simulink library "scp"  (R2021b)
settings: Solver=VariableStepAuto  StartTime=0.0  StopTime=10.0  RelTol=1e-3
undefined symbols (not defined in the file or in its folder): ENUM_ABSACTIVE_ACTIVE, ENUM_ABSACTIVE_INACTIVE, ENUM_ABSFAILED_FAILED, ENUM_ABSFAILED_NORMAL, ENUM_ABSFULLYOPER_FULLYOPER, ENUM_ABSFULLYOPER_INVALID, ENUM_ABSFULLYOPER_NOTFULLYOPER, ENUM_ABSFULLYOPER_RESERVED, ENUM_ABSWNLMPSTA_CONSTANT, ENUM_ABSWNLMPSTA_OFF, ENUM_AMBERWNLMPSTA_CONSTANT, ENUM_AMBERWNLMPSTA_OFF, ENUM_ANTILBRAKABSACT_ACTIVE, ENUM_ANTILBRAKABSACT_INVALID, ENUM_ANTILBRAKABSACT_PASSIVE, ENUM_ANTILBRAKABSACT_RESERVED, ENUM_BRKSWSTA_ACTIVE, ENUM_BRKSWSTA_INACTIVE, ENUM_EBSAMWARNLAMPSTA_NOACTION, ENUM_EBSAMWARNLAMPSTA_OFF, ENUM_EBSAMWARNLAMPSTA_ON, ENUM_EBSAMWARNLAMPSTA_RESERVED, ENUM_EBSBRAKESW_ERROR, ENUM_EBSBRAKESW_INVALID, ENUM_EBSBRAKESW_PRESSED, ENUM_EBSBRAKESW_UNPRESSED, ENUM_EBSREDWARNLAMPSTA_NOACTION, ENUM_EBSREDWARNLAMPSTA_OFF, ENUM_EBSREDWARNLAMPSTA_ON, ENUM_EBSREDWARNLAMPSTA_RESERVED, ENUM_FRDOORPOSISTA_CLOSED, ENUM_FRDOORPOSISTA_NODEFINE, ENUM_FRDOORPOSISTA_OPEN, ENUM_FRDOORPOSISTA_PARTIALOPEN, ENUM_HILLHOLDERMODE_ACTIVE, ENUM_HILLHOLDERMODE_ACTIVE2INACTIVE, ENUM_HILLHOLDERMODE_ACTIVEMAYPARK, ENUM_HILLHOLDERMODE_INACTIVE, ENUM_HILLHOLDERMODE_INVALID, ENUM_HILLHOLDERMODE_NOFUNC, ENUM_HILLHOLDERMODE_RESERVED4, ENUM_HILLHOLDERMODE_RESERVED5, ENUM_HSAACTIVE_ACTIVE, ENUM_HSAACTIVE_INACTIVE, ENUM_HSAFAILED_FAILED, ENUM_HSAFAILED_NORMAL, ENUM_OPENSTATUSOFDOOR1_CLOSED, ENUM_OPENSTATUSOFDOOR1_OPENED, ENUM_REDWNLMPSTA_CONSTANT, ENUM_REDWNLMPSTA_OFF, FALSE, KSCP_DelayECBAMandECDT_s, KSCP_DelayECDTandECDT_s, KSCP_DelayECDTandRCBAM_s, KSCP_DelayRCBAMandRCDT_s, KSCP_DelayRCDTandECBAM_s, KSCP_DelayRCDTandRCDT_s, KTQD_MCUMaxRefTq_Nm, TRUE
libraries: FVT_lib x14, hcu_lib x10, simulink x2
settings Model: Creator=FVT23118  LastModifiedBy=FVT22063

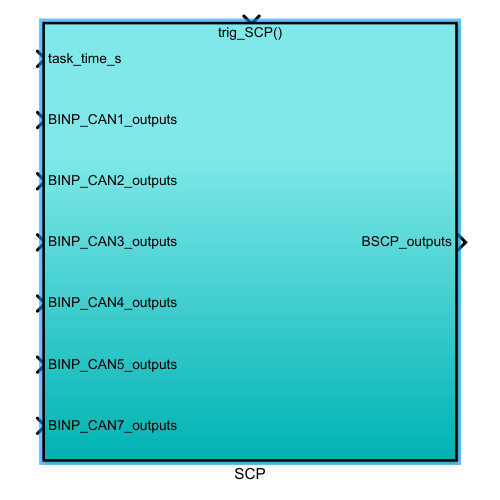
[thumbnail: Simulink's stored preview of the top-level diagram]
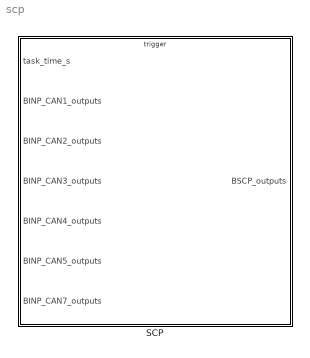
== system scp ==
  SCP : Subsystem
      settings: RTWSystemCode=Nonreusable function  RTWFcnNameOpts=Use subsystem name  RTWFileNameOpts=Use subsystem name

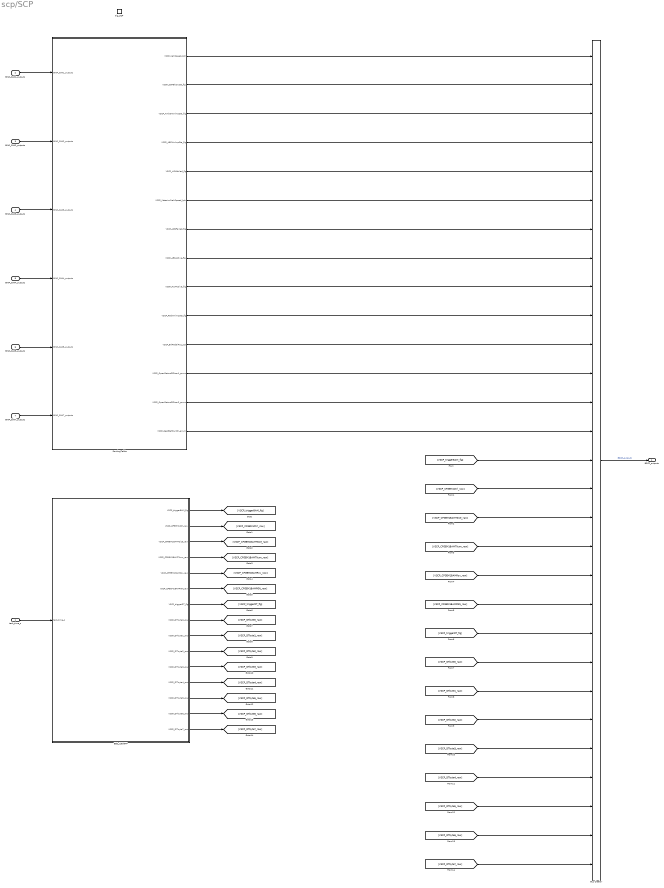
== system scp/SCP ==
  task_time_s : Inport
  BINP_CAN1_outputs : Inport  Port=2  OutDataTypeStr=Bus: BINP_CAN1_outputs
  BINP_CAN2_outputs : Inport  Port=3  OutDataTypeStr=Bus: BINP_CAN2_outputs
  BINP_CAN3_outputs : Inport  Port=4  OutDataTypeStr=Bus: BINP_CAN3_outputs
  BINP_CAN4_outputs : Inport  Port=5  OutDataTypeStr=Bus: BINP_CAN4_outputs
  BINP_CAN5_outputs : Inport  Port=6  OutDataTypeStr=Bus: BINP_CAN5_outputs
  BINP_CAN7_outputs : Inport  Port=7  OutDataTypeStr=Bus: BINP_CAN7_outputs
  trig_SCP : TriggerPort  TriggerType=function-call  VariantControl=(inherit)  PortDimensions=1
  Bus Creator : BusCreator  Inputs=29  OutDataTypeStr=Bus: BSCP_outputs  NonVirtualBus=on
  EBS_J1939TP : Subsystem
  RoutingTable : Subsystem
  BSCP_outputs : Outport  OutDataTypeStr=Bus: BSCP_outputs
  wires:
  BINP_CAN1_outputs/1 -> RoutingTable/1(BINP_CAN1_outputs)
  BINP_CAN4_outputs/1 -> RoutingTable/4(BINP_CAN4_outputs)
  BINP_CAN3_outputs/1 -> RoutingTable/3(BINP_CAN3_outputs)
  BINP_CAN2_outputs/1 -> RoutingTable/2(BINP_CAN2_outputs)
  BINP_CAN5_outputs/1 -> RoutingTable/5(BINP_CAN5_outputs)
  BINP_CAN7_outputs/1 -> RoutingTable/6(BINP_CAN7_outputs)
  RoutingTable/5(VSCP_HSAFailed_flg) -> Bus Creator/5
  RoutingTable/6(VSCP_MeterIndVehSpeed_kph) -> Bus Creator/6
  RoutingTable/4(VSCP_ABSWnlmpSta_flg) -> Bus Creator/4
  RoutingTable/7(VSCP_ABSFailed_flg) -> Bus Creator/7
  RoutingTable/3(VSCP_AmberWnlmpSta_flg) -> Bus Creator/3
  RoutingTable/8(VSCP_ABSActive_flg) -> Bus Creator/8
  RoutingTable/2(VSCP_SCPBrkSwSta_flg) -> Bus Creator/2
  RoutingTable/9(VSCP_HSAActive_flg) -> Bus Creator/9
  RoutingTable/1(VSCP_VehSpeed_kph) -> Bus Creator/1
  RoutingTable/10(VSCP_RedWnlmpSta_flg) -> Bus Creator/10
  RoutingTable/11(VSCP_BrkPedalPos_pct) -> Bus Creator/11
  RoutingTable/12(VSCP_OpenStatusOfDoor1_enum) -> Bus Creator/12
  RoutingTable/13(VSCP_OpenStatusOfDoor2_enum) -> Bus Creator/13
  RoutingTable/14(VSCP_SeatBeltSwitch_enum) -> Bus Creator/14
  Bus Creator/1 -> BSCP_outputs/1  "BSCP_outputs"
  EBS_J1939TP/1(VSCP_triggerBAM_flg) -> [VSCP_triggerBAM_flg]
  EBS_J1939TP/2(VSCP_CFGEM1Ctrl_raw) -> [VSCP_CFGEM1Ctrl_raw]
  EBS_J1939TP/3(VSCP_CFGEM1BAMTSize_raw) -> [VSCP_CFGEM1BAMTSize_raw]
  EBS_J1939TP/4(VSCP_CFGEM1BAMTNum_raw) -> [VSCP_CFGEM1BAMTNum_raw]
  EBS_J1939TP/5(VSCP_CFGEM1BAMRsv_raw) -> [VSCP_CFGEM1BAMRsv_raw]
  EBS_J1939TP/6(VSCP_CFGEM1BAMPGN_raw) -> [VSCP_CFGEM1BAMPGN_raw]
  EBS_J1939TP/7(VSCP_triggerDT_flg) -> [VSCP_triggerDT_flg]
  EBS_J1939TP/8(VSCP_DTbyte0_raw) -> [VSCP_DTbyte0_raw]
  EBS_J1939TP/9(VSCP_DTbyte1_raw) -> [VSCP_DTbyte1_raw]
  EBS_J1939TP/10(VSCP_DTbyte2_raw) -> [VSCP_DTbyte2_raw]
  EBS_J1939TP/11(VSCP_DTbyte3_raw) -> [VSCP_DTbyte3_raw]
  EBS_J1939TP/12(VSCP_DTbyte4_raw) -> [VSCP_DTbyte4_raw]
  EBS_J1939TP/13(VSCP_DTbyte5_raw) -> [VSCP_DTbyte5_raw]
  EBS_J1939TP/14(VSCP_DTbyte6_raw) -> [VSCP_DTbyte6_raw]
  EBS_J1939TP/15(VSCP_DTbyte7_raw) -> [VSCP_DTbyte7_raw]
  [VSCP_DTbyte7_raw] -> Bus Creator/29
  [VSCP_DTbyte6_raw] -> Bus Creator/28
  [VSCP_DTbyte5_raw] -> Bus Creator/27
  [VSCP_DTbyte4_raw] -> Bus Creator/26
  [VSCP_DTbyte3_raw] -> Bus Creator/25
  [VSCP_DTbyte2_raw] -> Bus Creator/24
  [VSCP_DTbyte1_raw] -> Bus Creator/23
  [VSCP_DTbyte0_raw] -> Bus Creator/22
  [VSCP_triggerDT_flg] -> Bus Creator/21
  [VSCP_CFGEM1BAMPGN_raw] -> Bus Creator/20
  [VSCP_CFGEM1BAMRsv_raw] -> Bus Creator/19
  [VSCP_CFGEM1BAMTNum_raw] -> Bus Creator/18
  [VSCP_CFGEM1BAMTSize_raw] -> Bus Creator/17
  [VSCP_CFGEM1Ctrl_raw] -> Bus Creator/16
  [VSCP_triggerBAM_flg] -> Bus Creator/15
  task_time_s/1 -> EBS_J1939TP/1(task_time_s)

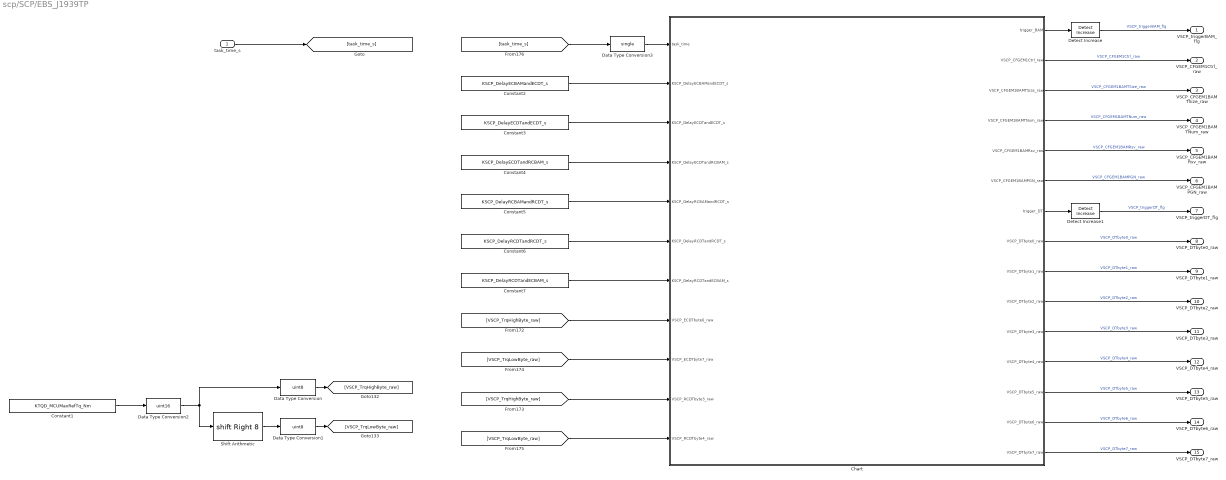
== system scp/SCP/EBS_J1939TP ==
  task_time_s : Inport
  Chart : Stateflow chart  TreatAsAtomicUnit=on
  Constant1 : Constant  Value=KTQD_MCUMaxRefTq_Nm
  Constant2 : Constant  Value=KSCP_DelayECBAMandECDT_s
  Constant3 : Constant  Value=KSCP_DelayECDTandECDT_s
  Constant4 : Constant  Value=KSCP_DelayECDTandRCBAM_s
  Constant5 : Constant  Value=KSCP_DelayRCBAMandRCDT_s
  Constant6 : Constant  Value=KSCP_DelayRCDTandRCDT_s
  Constant7 : Constant  Value=KSCP_DelayRCDTandECBAM_s
  Data Type Conversion : DataTypeConversion  OutDataTypeStr=uint8
  Data Type Conversion1 : DataTypeConversion  OutDataTypeStr=uint8
  Data Type Conversion2 : DataTypeConversion  OutDataTypeStr=uint16
  Data Type Conversion3 : DataTypeConversion  OutDataTypeStr=single
  Detect Increase : simulink/Logic and Bit Operations/Detect Increase  vinit=0.0  OutDataTypeStr=boolean
  Detect Increase1 : simulink/Logic and Bit Operations/Detect Increase  vinit=0.0  OutDataTypeStr=boolean
  Shift Arithmetic : ArithShift  BitShiftNumber=8  BitShiftDirection=Right
  VSCP_triggerBAM_flg : Outport
  VSCP_CFGEM1Ctrl_raw : Outport  Port=2
  VSCP_CFGEM1BAMTSize_raw : Outport  Port=3
  VSCP_CFGEM1BAMTNum_raw : Outport  Port=4
  VSCP_CFGEM1BAMRsv_raw : Outport  Port=5
  VSCP_CFGEM1BAMPGN_raw : Outport  Port=6
  VSCP_triggerDT_flg : Outport  Port=7
  VSCP_DTbyte0_raw : Outport  Port=8
  VSCP_DTbyte1_raw : Outport  Port=9
  VSCP_DTbyte2_raw : Outport  Port=10
  VSCP_DTbyte3_raw : Outport  Port=11
  VSCP_DTbyte4_raw : Outport  Port=12
  VSCP_DTbyte5_raw : Outport  Port=13
  VSCP_DTbyte6_raw : Outport  Port=14
  VSCP_DTbyte7_raw : Outport  Port=15
  wires:
  Constant2/1 -> Chart/2(KSCP_DelayECBAMandECDT_s)
  [task_time_s] -> Data Type Conversion3/1
  Data Type Conversion1/1 -> [VSCP_TrqLowByte_raw]
  [VSCP_TrqHighByte_raw] -> Chart/10(VSCP_RCDTbyte3_raw)
  [VSCP_TrqHighByte_raw] -> Chart/8(VSCP_ECDTbyte6_raw)
  Constant4/1 -> Chart/4(KSCP_DelayECDTandRCBAM_s)
  [VSCP_TrqLowByte_raw] -> Chart/11(VSCP_RCDTbyte4_raw)
  Constant1/1 -> Data Type Conversion2/1
  Constant5/1 -> Chart/5(KSCP_DelayRCBAMandRCDT_s)
  Data Type Conversion2/1 -> Data Type Conversion/1, Shift Arithmetic/1
  Shift Arithmetic/1 -> Data Type Conversion1/1
  Constant3/1 -> Chart/3(KSCP_DelayECDTandECDT_s)
  Constant6/1 -> Chart/6(KSCP_DelayRCDTandRCDT_s)
  Data Type Conversion/1 -> [VSCP_TrqHighByte_raw]
  [VSCP_TrqLowByte_raw] -> Chart/9(VSCP_ECDTbyte7_raw)
  Constant7/1 -> Chart/7(KSCP_DelayRCDTandECBAM_s)
  Chart/1(trigger_BAM) -> Detect Increase/1
  Chart/7(trigger_DT) -> Detect Increase1/1
  Detect Increase/1 -> VSCP_triggerBAM_flg/1  "VSCP_triggerBAM_flg"
  Chart/2(VSCP_CFGEM1Ctrl_raw) -> VSCP_CFGEM1Ctrl_raw/1  "VSCP_CFGEM1Ctrl_raw"
  Chart/3(VSCP_CFGEM1BAMTSize_raw) -> VSCP_CFGEM1BAMTSize_raw/1  "VSCP_CFGEM1BAMTSize_raw"
  Chart/4(VSCP_CFGEM1BAMTNum_raw) -> VSCP_CFGEM1BAMTNum_raw/1  "VSCP_CFGEM1BAMTNum_raw"
  Chart/5(VSCP_CFGEM1BAMRsv_raw) -> VSCP_CFGEM1BAMRsv_raw/1  "VSCP_CFGEM1BAMRsv_raw"
  Chart/6(VSCP_CFGEM1BAMPGN_raw) -> VSCP_CFGEM1BAMPGN_raw/1  "VSCP_CFGEM1BAMPGN_raw"
  Detect Increase1/1 -> VSCP_triggerDT_flg/1  "VSCP_triggerDT_flg"
  Chart/8(VSCP_DTbyte0_raw) -> VSCP_DTbyte0_raw/1  "VSCP_DTbyte0_raw"
  Chart/9(VSCP_DTbyte1_raw) -> VSCP_DTbyte1_raw/1  "VSCP_DTbyte1_raw"
  Chart/10(VSCP_DTbyte2_raw) -> VSCP_DTbyte2_raw/1  "VSCP_DTbyte2_raw"
  Chart/11(VSCP_DTbyte3_raw) -> VSCP_DTbyte3_raw/1  "VSCP_DTbyte3_raw"
  Chart/12(VSCP_DTbyte4_raw) -> VSCP_DTbyte4_raw/1  "VSCP_DTbyte4_raw"
  Chart/13(VSCP_DTbyte5_raw) -> VSCP_DTbyte5_raw/1  "VSCP_DTbyte5_raw"
  Chart/14(VSCP_DTbyte6_raw) -> VSCP_DTbyte6_raw/1  "VSCP_DTbyte6_raw"
  Chart/15(VSCP_DTbyte7_raw) -> VSCP_DTbyte7_raw/1  "VSCP_DTbyte7_raw"
  task_time_s/1 -> [task_time_s]
  Data Type Conversion3/1 -> Chart/1(task_time)

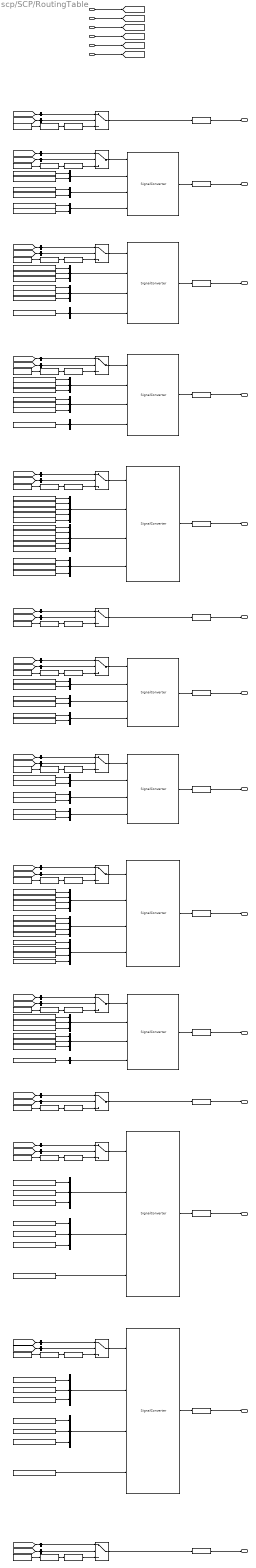
== system scp/SCP/RoutingTable ==
  BINP_CAN1_outputs : Inport
  BINP_CAN2_outputs : Inport  Port=2
  BINP_CAN3_outputs : Inport  Port=3
  BINP_CAN4_outputs : Inport  Port=4
  BINP_CAN5_outputs : Inport  Port=5
  BINP_CAN7_outputs : Inport  Port=6
  Constant : Constant  Value=ENUM_EBSBRAKESW_UNPRESSED
  Constant1 : Constant  Value=ENUM_EBSBRAKESW_PRESSED
  Constant10 : Constant  Value=ENUM_ABSFULLYOPER_RESERVED
  Constant11 : Constant  Value=ENUM_ABSWNLMPSTA_OFF
  Constant12 : Constant  Value=ENUM_ABSFULLYOPER_INVALID
  Constant13 : Constant  Value=ENUM_ABSWNLMPSTA_OFF
  Constant14 : Constant  Value=ENUM_AMBERWNLMPSTA_OFF
  Constant15 : Constant  Value=ENUM_EBSAMWARNLAMPSTA_NOACTION
  Constant16 : Constant  Value=ENUM_AMBERWNLMPSTA_CONSTANT
  Constant17 : Constant  Value=ENUM_EBSAMWARNLAMPSTA_OFF
  Constant18 : Constant  Value=ENUM_EBSAMWARNLAMPSTA_ON
  Constant19 : Constant  Value=ENUM_AMBERWNLMPSTA_OFF
  Constant2 : Constant  Value=ENUM_BRKSWSTA_INACTIVE
  Constant20 : Constant  Value=ENUM_HILLHOLDERMODE_RESERVED4
  Constant{21,23,26,29} (4 alike) : Constant  Value=ENUM_HSAFAILED_NORMAL
  Constant22 : Constant  Value=ENUM_HILLHOLDERMODE_ACTIVE2INACTIVE
  Constant24 : Constant  Value=ENUM_HILLHOLDERMODE_INACTIVE
  Constant25 : Constant  Value=ENUM_HILLHOLDERMODE_ACTIVE
  Constant27 : Constant  Value=ENUM_HILLHOLDERMODE_NOFUNC
  Constant28 : Constant  Value=ENUM_HILLHOLDERMODE_ACTIVEMAYPARK
  Constant3 : Constant  Value=ENUM_BRKSWSTA_ACTIVE
  Constant30 : Constant  Value=ENUM_HSAFAILED_FAILED
  Constant31 : Constant  Value=ENUM_HILLHOLDERMODE_RESERVED5
  Constant32 : Constant  Value=ENUM_HILLHOLDERMODE_INVALID
  Constant33 : Constant  Value=ENUM_ABSFULLYOPER_RESERVED
  Constant34 : Constant  Value=ENUM_ABSFULLYOPER_INVALID
  Constant35 : Constant  Value=ENUM_ANTILBRAKABSACT_RESERVED
  Constant36 : Constant  Value=ENUM_ABSFAILED_NORMAL
  Constant37 : Constant  Value=ENUM_ABSFULLYOPER_NOTFULLYOPER
  Constant38 : Constant  Value=ENUM_ABSFULLYOPER_FULLYOPER
  Constant39 : Constant  Value=ENUM_ABSFAILED_FAILED
  Constant4 : Constant  Value=ENUM_EBSBRAKESW_ERROR
  Constant40 : Constant  Value=ENUM_ANTILBRAKABSACT_INVALID
  Constant41 : Constant  Value=ENUM_ABSACTIVE_ACTIVE
  Constant42 : Constant  Value=ENUM_ANTILBRAKABSACT_PASSIVE
  Constant43 : Constant  Value=ENUM_ANTILBRAKABSACT_ACTIVE
  Constant44 : Constant  Value=ENUM_ABSACTIVE_INACTIVE
  Constant45 : Constant  Value=ENUM_HILLHOLDERMODE_RESERVED4
  Constant46 : Constant  Value=ENUM_HSAACTIVE_INACTIVE
  Constant47 : Constant  Value=ENUM_HILLHOLDERMODE_ACTIVE2INACTIVE
  Constant48 : Constant  Value=ENUM_HSAACTIVE_ACTIVE
  Constant49 : Constant  Value=ENUM_HILLHOLDERMODE_INACTIVE
  Constant5 : Constant  Value=ENUM_EBSBRAKESW_INVALID
  Constant50 : Constant  Value=ENUM_HILLHOLDERMODE_ACTIVE
  Constant51 : Constant  Value=ENUM_HSAACTIVE_ACTIVE
  Constant52 : Constant  Value=ENUM_HILLHOLDERMODE_NOFUNC
  Constant53 : Constant  Value=ENUM_HILLHOLDERMODE_ACTIVEMAYPARK
  Constant54 : Constant  Value=ENUM_HSAACTIVE_ACTIVE
  Constant55 : Constant  Value=ENUM_EBSREDWARNLAMPSTA_RESERVED
  Constant56 : Constant  Value=ENUM_HILLHOLDERMODE_RESERVED5
  Constant57 : Constant  Value=ENUM_HILLHOLDERMODE_INVALID
  Constant58 : Constant  Value=ENUM_EBSREDWARNLAMPSTA_NOACTION
  Constant59 : Constant  Value=ENUM_REDWNLMPSTA_CONSTANT
  Constant6 : Constant  Value=ENUM_ABSFULLYOPER_NOTFULLYOPER
  Constant60 : Constant  Value=ENUM_EBSREDWARNLAMPSTA_OFF
  Constant61 : Constant  Value=ENUM_EBSREDWARNLAMPSTA_ON
  Constant62 : Constant  Value=ENUM_REDWNLMPSTA_OFF
  Constant63 : Constant  Value=ENUM_REDWNLMPSTA_OFF
  Constant64 : Constant  Value=ENUM_FRDOORPOSISTA_NODEFINE
  Constant65 : Constant  Value=ENUM_OPENSTATUSOFDOOR1_CLOSED
  Constant66 : Constant  Value=ENUM_FRDOORPOSISTA_PARTIALOPEN
  Constant{67,70,74,77} (4 alike) : Constant  Value=ENUM_OPENSTATUSOFDOOR1_OPENED
  Constant68 : Constant  Value=ENUM_FRDOORPOSISTA_CLOSED
  Constant69 : Constant  Value=ENUM_FRDOORPOSISTA_OPEN
  Constant7 : Constant  Value=ENUM_ABSFULLYOPER_FULLYOPER
  Constant71 : Constant  Value=ENUM_FRDOORPOSISTA_NODEFINE
  Constant72 : Constant  Value=ENUM_OPENSTATUSOFDOOR1_CLOSED
  Constant73 : Constant  Value=ENUM_FRDOORPOSISTA_PARTIALOPEN
  Constant75 : Constant  Value=ENUM_FRDOORPOSISTA_CLOSED
  Constant76 : Constant  Value=ENUM_FRDOORPOSISTA_OPEN
  Constant8 : Constant  Value=ENUM_EBSAMWARNLAMPSTA_RESERVED
  Constant9 : Constant  Value=ENUM_ABSWNLMPSTA_CONSTANT
  Mux{,1..2,12..17} (9 alike) : Mux  Inputs=2
  Mux10 : Mux  Inputs=5
  Mux{3..4,6..7,11,21,23..27} (11 alike) : Mux  Inputs=3
  Mux18 : Mux
  Mux19 : Mux
  Mux20 : Mux
  Mux22 : Mux  Inputs=1
  Mux5 : Mux  Inputs=1
  Mux8 : Mux  Inputs=1
  Mux9 : Mux  Inputs=5
  SignalConverter{1..3,5..6,8} (6 alike) : hcu_lib/Basic_Blocks/SignalConverter  SourceSignalInitialValue=0  SourceSignalUpperLimit=3  SourceSignalLowerLimit=0  ConvertedSignalInitialValue=0
  SignalConverter10 : hcu_lib/Basic_Blocks/SignalConverter  SourceSignalInitialValue=0  SourceSignalUpperLimit=15  SourceSignalLowerLimit=0  ConvertedSignalInitialValue=0
  SignalConverter4 : hcu_lib/Basic_Blocks/SignalConverter  SourceSignalInitialValue=0  SourceSignalUpperLimit=7  SourceSignalLowerLimit=0  ConvertedSignalInitialValue=0
  SignalConverter7 : hcu_lib/Basic_Blocks/SignalConverter  SourceSignalInitialValue=0  SourceSignalUpperLimit=7  SourceSignalLowerLimit=0  ConvertedSignalInitialValue=0
  SignalConverter9 : hcu_lib/Basic_Blocks/SignalConverter  SourceSignalInitialValue=0  SourceSignalUpperLimit=15  SourceSignalLowerLimit=0  ConvertedSignalInitialValue=0
  convert{1,4,11..12,21..22} (6 alike) : DataTypeConversion  OutDataTypeStr=single
  convert{3,6,8,10,14,16..17,20,27} (9 alike) : DataTypeConversion  OutDataTypeStr=boolean
  convert{2,5,7,9,13,15,18..19,23..26,28} (13 alike) : DataTypeConversion  OutDataTypeStr=uint8
  convert_in : FVT_lib/hal/convert_in  gain=0.00390625  offset=0
  convert_in{1..4,6..9,11..13} (11 alike) : FVT_lib/hal/convert_in  gain=1  offset=0
  convert_in10 : FVT_lib/hal/convert_in  gain=0.4  offset=0
  convert_in5 : FVT_lib/hal/convert_in  gain=0.00390625  offset=0
  cst_1 : Constant  Value=0xFB00
  cst_{2..5,7..11,14} (10 alike) : Constant  Value=0x0
  cst_12 : Constant  Value=0x3
  cst_13 : Constant  Value=0x3
  cst_6 : Constant  Value=0xFB00
  slr2_1 : BusSelector  OutputSignals=VINP_CANMsgValidEBC2_flg
  slr2_{2..4,7..8,10..11} (7 alike) : BusSelector  OutputSignals=VINP_CANMsgValidEBC1_flg
  slr2_12 : BusSelector  OutputSignals=VINP_CANMsgValidDoorFr1_flg
  slr2_13 : BusSelector  OutputSignals=VINP_CANMsgValidDoorFr1_flg
  slr2_14 : BusSelector  OutputSignals=VINP_CANMsgValidZ24CE1000_flg
  slr2_5 : BusSelector  OutputSignals=VINP_CANMsgValidEBC5_flg
  slr2_6 : BusSelector  OutputSignals=VINP_CANMsgValidEBC2_flg
  slr2_9 : BusSelector  OutputSignals=VINP_CANMsgValidEBC5_flg
  slr_1 : BusSelector  OutputSignals=VINP_FASpeed_kph
  slr_10 : BusSelector  OutputSignals=VINP_EBSRedWarnLampSta_enum
  slr_11 : BusSelector  OutputSignals=VINP_BrakePedalPos_pct
  slr_12 : BusSelector  OutputSignals=VINP_DoorFrDoorpositionsta_enum
  slr_13 : BusSelector  OutputSignals=VINP_DoorFrDoorpositionsta_enum
  slr_14 : BusSelector  OutputSignals=VINP_Z24BCMSeatBeltSWSta_flg
  slr_2 : BusSelector  OutputSignals=VINP_EBSBrakeSw_enum
  slr_3 : BusSelector  OutputSignals=VINP_EBSAmWarnLampSta_enum
  slr_4 : BusSelector  OutputSignals=VINP_ABSFullyOper_enum
  slr_5 : BusSelector  OutputSignals=VINP_HillHolderMode_enum
  slr_6 : BusSelector  OutputSignals=VINP_FASpeed_kph
  slr_7 : BusSelector  OutputSignals=VINP_ABSFullyOper_enum
  slr_8 : BusSelector  OutputSignals=VINP_AntiLBrakABSAct_enum
  slr_9 : BusSelector  OutputSignals=VINP_HillHolderMode_enum
  sw_{1..14} (14 alike) : Switch  Criteria=u2 > Threshold
  VSCP_VehSpeed_kph : Outport
  VSCP_SCPBrkSwSta_flg : Outport  Port=2
  VSCP_AmberWnlmpSta_flg : Outport  Port=3
  VSCP_ABSWnlmpSta_flg : Outport  Port=4
  VSCP_HSAFailed_flg : Outport  Port=5
  VSCP_MeterIndVehSpeed_kph : Outport  Port=6
  VSCP_ABSFailed_flg : Outport  Port=7
  VSCP_ABSActive_flg : Outport  Port=8
  VSCP_HSAActive_flg : Outport  Port=9
  VSCP_RedWnlmpSta_flg : Outport  Port=10
  VSCP_BrkPedalPos_pct : Outport  Port=11
  VSCP_OpenStatusOfDoor1_enum : Outport  Port=12
  VSCP_OpenStatusOfDoor2_enum : Outport  Port=13
  VSCP_SeatBeltSwitch_enum : Outport  Port=14
  wires:
  BINP_CAN1_outputs/1 -> [BINP_CAN1_outputs]
  BINP_CAN2_outputs/1 -> [BINP_CAN2_outputs]
  BINP_CAN3_outputs/1 -> [BINP_CAN3_outputs]
  BINP_CAN4_outputs/1 -> [BINP_CAN4_outputs]
  BINP_CAN5_outputs/1 -> [BINP_CAN5_outputs]
  [BINP_CAN1_outputs] -> slr_1/1
  [BINP_CAN1_outputs] -> slr2_1/1
  cst_1/1 -> convert_in/1
  convert_in/1 -> convert1/1
  convert1/1 -> sw_1/3
  sw_1/1 -> convert4/1
  convert2/1 -> sw_2/3
  convert_in1/1 -> convert2/1
  cst_2/1 -> convert_in1/1
  [BINP_CAN1_outputs] -> slr2_2/1
  [BINP_CAN1_outputs] -> slr_2/1
  sw_2/1 -> SignalConverter1/1
  SignalConverter1/1 -> convert3/1
  Mux/1 -> SignalConverter1/2
  Constant/1 -> Mux/1
  Constant1/1 -> Mux/2
  Constant3/1 -> Mux1/2
  Constant2/1 -> Mux1/1
  Mux1/1 -> SignalConverter1/3
  Mux2/1 -> SignalConverter1/4
  Constant4/1 -> Mux2/1
  Constant5/1 -> Mux2/2
  convert3/1 -> VSCP_SCPBrkSwSta_flg/1  "VSCP_SCPBrkSwSta_flg"
  convert4/1 -> VSCP_VehSpeed_kph/1  "VSCP_Vehspeed_kph"
  convert6/1 -> VSCP_AmberWnlmpSta_flg/1  "VSCP_AmberWnlmpSta_flg"
  Constant10/1 -> Mux5/1
  Constant7/1 -> Mux3/2
  Constant6/1 -> Mux3/1
  SignalConverter2/1 -> convert6/1
  sw_3/1 -> SignalConverter2/1
  [BINP_CAN1_outputs] -> slr_3/1
  [BINP_CAN1_outputs] -> slr2_3/1
  cst_3/1 -> convert_in2/1
  convert_in2/1 -> convert5/1
  convert5/1 -> sw_3/3
  Constant12/1 -> Mux3/3
  Constant11/1 -> Mux4/3
  Constant9/1 -> Mux4/1
  Constant13/1 -> Mux4/2
  slr_1/1 -> sw_1/1  "<VINP_FASpeed_kph>"
  slr2_1/1 -> sw_1/2  "<VINP_CANMsgValidEBC2_flg>"
  slr2_2/1 -> sw_2/2  "<VINP_CANMsgValidEBC1_flg>"
  slr_2/1 -> sw_2/1  "<VINP_EBSBrakeSw_enum>"
  slr2_3/1 -> sw_3/2  "<VINP_CANMsgValidEBC1_flg>"
  slr_3/1 -> sw_3/1  "<VINP_EBSAmWarnLampSta_enum>"
  slr_4/1 -> sw_4/1  "<VINP_ABSFullyOper_enum>"
  slr2_4/1 -> sw_4/2  "<VINP_CANMsgValidEBC1_flg>"
  Constant16/1 -> Mux7/2
  Constant19/1 -> Mux7/1
  Constant14/1 -> Mux7/3
  Constant15/1 -> Mux6/3
  convert7/1 -> sw_4/3
  convert_in3/1 -> convert7/1
  cst_4/1 -> convert_in3/1
  [BINP_CAN1_outputs] -> slr2_4/1
  [BINP_CAN1_outputs] -> slr_4/1
  sw_4/1 -> SignalConverter3/1
  SignalConverter3/1 -> convert8/1
  Constant17/1 -> Mux6/1
  Constant18/1 -> Mux6/2
  Constant8/1 -> Mux8/1
  convert8/1 -> VSCP_ABSWnlmpSta_flg/1  "VSCP_ABSWnlmpSta_flg"
  Mux6/1 -> SignalConverter2/2
  Mux7/1 -> SignalConverter2/3
  Mux8/1 -> SignalConverter2/4
  Mux3/1 -> SignalConverter3/2
  Mux4/1 -> SignalConverter3/3
  Mux5/1 -> SignalConverter3/4
  Mux11/1 -> SignalConverter4/4
  Mux9/1 -> SignalConverter4/2
  convert10/1 -> VSCP_HSAFailed_flg/1  "VSCP_HSAFailed_flg"
  SignalConverter4/1 -> convert10/1
  sw_5/1 -> SignalConverter4/1
  [BINP_CAN1_outputs] -> slr_5/1
  [BINP_CAN1_outputs] -> slr2_5/1
  cst_5/1 -> convert_in4/1
  convert_in4/1 -> convert9/1
  convert9/1 -> sw_5/3
  slr2_5/1 -> sw_5/2  "<VINP_CANMsgValidEBC5_flg>"
  slr_5/1 -> sw_5/1  "<VINP_HillHolderMode_enum>"
  Constant22/1 -> Mux9/3
  Constant24/1 -> Mux9/1
  Constant25/1 -> Mux9/2
  Constant20/1 -> Mux11/1
  Constant28/1 -> Mux9/4
  Constant27/1 -> Mux9/5
  Constant30/1 -> Mux10/5
  Constant29/1 -> Mux10/4
  Constant23/1 -> Mux10/2
  Constant21/1 -> Mux10/1
  Constant26/1 -> Mux10/3
  Mux10/1 -> SignalConverter4/3
  Constant31/1 -> Mux11/2
  Constant32/1 -> Mux11/3
  convert_in5/1 -> convert11/1
  convert12/1 -> VSCP_MeterIndVehSpeed_kph/1  "VSCP_MeterIndVehSpeed_kph"
  [BINP_CAN1_outputs] -> slr_6/1
  [BINP_CAN1_outputs] -> slr2_6/1
  convert11/1 -> sw_6/3
  cst_6/1 -> convert_in5/1
  slr_6/1 -> sw_6/1  "<VINP_FASpeed_kph>"
  sw_6/1 -> convert12/1
  slr2_6/1 -> sw_6/2  "<VINP_CANMsgValidEBC2_flg>"
  Constant36/1 -> Mux15/2
  Constant39/1 -> Mux15/1
  Constant37/1 -> Mux12/1
  Constant38/1 -> Mux12/2
  Mux15/1 -> SignalConverter5/3
  Mux12/1 -> SignalConverter5/2
  convert14/1 -> VSCP_ABSFailed_flg/1  "VSCP_ABSFailed_flg"
  SignalConverter5/1 -> convert14/1
  sw_7/1 -> SignalConverter5/1
  [BINP_CAN1_outputs] -> slr2_7/1
  [BINP_CAN1_outputs] -> slr_7/1
  convert_in6/1 -> convert13/1
  convert13/1 -> sw_7/3
  slr2_7/1 -> sw_7/2  "<VINP_CANMsgValidEBC1_flg>"
  slr_7/1 -> sw_7/1  "<VINP_ABSFullyOper_enum>"
  cst_7/1 -> convert_in6/1
  Mux13/1 -> SignalConverter5/4
  Constant33/1 -> Mux13/1
  Constant34/1 -> Mux13/2
  Constant40/1 -> Mux16/2
  Constant35/1 -> Mux16/1
  Mux16/1 -> SignalConverter6/4
  cst_8/1 -> convert_in7/1
  slr_8/1 -> sw_8/1  "<VINP_AntiLBrakABSAct_enum>"
  slr2_8/1 -> sw_8/2  "<VINP_CANMsgValidEBC1_flg>"
  convert15/1 -> sw_8/3
  convert_in7/1 -> convert15/1
  [BINP_CAN1_outputs] -> slr_8/1
  [BINP_CAN1_outputs] -> slr2_8/1
  sw_8/1 -> SignalConverter6/1
  SignalConverter6/1 -> convert16/1
  convert16/1 -> VSCP_ABSActive_flg/1  "VSCP_ABSActive_flg"
  Mux14/1 -> SignalConverter6/2
  Mux17/1 -> SignalConverter6/3
  Constant43/1 -> Mux14/2
  Constant42/1 -> Mux14/1
  Constant44/1 -> Mux17/1
  Constant41/1 -> Mux17/2
  Constant57/1 -> Mux19/3
  Constant56/1 -> Mux19/2
  Mux18/1 -> SignalConverter7/3
  Constant51/1 -> Mux18/3
  Constant46/1 -> Mux18/1
  Constant48/1 -> Mux18/2
  Constant54/1 -> Mux18/4
  Constant52/1 -> Mux19/4
  Constant53/1 -> Mux20/4
  Constant45/1 -> Mux19/1
  Constant50/1 -> Mux20/2
  Constant49/1 -> Mux20/1
  Constant47/1 -> Mux20/3
  slr_9/1 -> sw_9/1  "<VINP_HillHolderMode_enum>"
  slr2_9/1 -> sw_9/2  "<VINP_CANMsgValidEBC5_flg>"
  convert18/1 -> sw_9/3
  convert_in8/1 -> convert18/1
  cst_9/1 -> convert_in8/1
  [BINP_CAN1_outputs] -> slr2_9/1
  [BINP_CAN1_outputs] -> slr_9/1
  sw_9/1 -> SignalConverter7/1
  SignalConverter7/1 -> convert17/1
  convert17/1 -> VSCP_HSAActive_flg/1  "VSCP_HSAActive_flg"
  Mux20/1 -> SignalConverter7/2
  Mux19/1 -> SignalConverter7/4
  Constant59/1 -> Mux23/2
  Constant62/1 -> Mux23/1
  Constant60/1 -> Mux21/1
  Constant61/1 -> Mux21/2
  Mux23/1 -> SignalConverter8/3
  Mux21/1 -> SignalConverter8/2
  convert20/1 -> VSCP_RedWnlmpSta_flg/1  "VSCP_RedWnlmpSta_flg"
  SignalConverter8/1 -> convert20/1
  sw_10/1 -> SignalConverter8/1
  [BINP_CAN1_outputs] -> slr2_10/1
  [BINP_CAN1_outputs] -> slr_10/1
  convert_in9/1 -> convert19/1
  convert19/1 -> sw_10/3
  slr2_10/1 -> sw_10/2  "<VINP_CANMsgValidEBC1_flg>"
  slr_10/1 -> sw_10/1  "<VINP_EBSRedWarnLampSta_enum>"
  cst_10/1 -> convert_in9/1
  Mux22/1 -> SignalConverter8/4
  Constant55/1 -> Mux22/1
  Constant58/1 -> Mux21/3
  Constant63/1 -> Mux23/3
  sw_11/1 -> convert22/1
  convert21/1 -> sw_11/3
  cst_11/1 -> convert_in10/1
  convert22/1 -> VSCP_BrkPedalPos_pct/1  "VSCP_BrkPedalPos_pct"
  convert_in10/1 -> convert21/1
  BINP_CAN7_outputs/1 -> [BINP_CAN7_outputs]
  [BINP_CAN7_outputs] -> slr_12/1
  slr_11/1 -> sw_11/1  "<VINP_BrakePedalPos_pct>"
  slr2_11/1 -> sw_11/2  "<VINP_CANMsgValidEBC1_flg>"
  [BINP_CAN1_outputs] -> slr_11/1
  [BINP_CAN1_outputs] -> slr2_11/1
  Constant68/1 -> Mux26/1
  convert_in11/1 -> convert24/1
  convert24/1 -> sw_12/3
  cst_12/1 -> convert_in11/1
  convert23/1 -> VSCP_OpenStatusOfDoor1_enum/1  "VSCP_OpenStatusOfDoor1_enum"
  Constant64/1 -> SignalConverter9/4
  Mux26/1 -> SignalConverter9/2
  sw_12/1 -> SignalConverter9/1
  SignalConverter9/1 -> convert23/1
  Mux24/1 -> SignalConverter9/3
  Constant69/1 -> Mux26/2
  Constant67/1 -> Mux24/2
  Constant65/1 -> Mux24/1
  Constant66/1 -> Mux26/3
  Constant70/1 -> Mux24/3
  [BINP_CAN7_outputs] -> slr2_12/1
  slr_12/1 -> sw_12/1  "<VINP_DoorFrDoorpositionsta_enum>"
  slr2_12/1 -> sw_12/2  "<VINP_CANMsgValidDoorFr1_flg>"
  SignalConverter10/1 -> convert25/1
  convert25/1 -> VSCP_OpenStatusOfDoor2_enum/1  "VSCP_OpenStatusOfDoor2_enum"
  slr2_14/1 -> sw_14/2  "<VINP_CANMsgValidZ24CE1000_flg>"
  sw_14/1 -> convert28/1
  slr_14/1 -> sw_14/1  "<VINP_Z24BCMSeatBeltSWSta_flg>"
  cst_14/1 -> convert_in13/1
  convert27/1 -> sw_14/3
  [BINP_CAN4_outputs] -> slr2_14/1
  [BINP_CAN4_outputs] -> slr_14/1
  convert28/1 -> VSCP_SeatBeltSwitch_enum/1  "VSCP_SeatBeltSwitch_enum"
  convert_in13/1 -> convert27/1
  convert_in12/1 -> convert26/1
  sw_13/1 -> SignalConverter10/1
  slr_13/1 -> sw_13/1  "<VINP_DoorFrDoorpositionsta_enum>"
  [BINP_CAN7_outputs] -> slr2_13/1
  cst_13/1 -> convert_in12/1
  slr2_13/1 -> sw_13/2  "<VINP_CANMsgValidDoorFr1_flg>"
  convert26/1 -> sw_13/3
  [BINP_CAN7_outputs] -> slr_13/1
  Constant77/1 -> Mux25/3
  Constant76/1 -> Mux27/2
  Constant72/1 -> Mux25/1
  Constant75/1 -> Mux27/1
  Constant74/1 -> Mux25/2
  Mux27/1 -> SignalConverter10/2
  Mux25/1 -> SignalConverter10/3
  Constant71/1 -> SignalConverter10/4
  Constant73/1 -> Mux27/3

== stateflow chart scp/SCP/EBS_J1939TP/Chart ==
  state TP
    state Trigger_ECBAM_and_Delay
      en: trigger_BAM = TRUE;
      (default) -> (junction 21) : {
          |  VSCP_TpDelayDone_flg = FALSE;
          |  VSCP_TimeTPdelay_s = 0;
          | }
      Trigger_ECBAM_and_Delay -> (junction 21) [order 1] : {trigger_BAM = FALSE;}
      (junction 21) -> (junction 26) [order 1] : [VSCP_TimeTPdelay_s >= KSCP_DelayECBAMandECDT_s]
      (junction 21) -> (junction 24) [order 2] : {VSCP_TimeTPdelay_s += task_time;}
      (junction 26) -> (junction 28) : {VSCP_TpDelayDone_flg = TRUE;}
      (junction 28) -> (junction 24)
    state Tirgger_ECDT1_and_Delay
      en: trigger_DT = TRUE;
      (default) -> (junction 32) : {
          |  VSCP_TpDelayDone_flg = FALSE;
          |  VSCP_TimeTPdelay_s = 0;}
      Tirgger_ECDT1_and_Delay -> (junction 32) [order 1] : {trigger_DT = FALSE;}
      (junction 32) -> (junction 33) [order 1] : [VSCP_TimeTPdelay_s >= KSCP_DelayECDTandECDT_s]
      (junction 32) -> (junction 34) [order 2] : {VSCP_TimeTPdelay_s += task_time;}
      (junction 33) -> (junction 35) : {VSCP_TpDelayDone_flg = TRUE;}
      (junction 35) -> (junction 34)
    state Tirgger_ECDT2_and_Delay
      en: trigger_DT = TRUE;
      (default) -> (junction 55) : {
          |  VSCP_TpDelayDone_flg = FALSE;
          |  VSCP_TimeTPdelay_s = 0;}
      Tirgger_ECDT2_and_Delay -> (junction 55) [order 1] : {trigger_DT = FALSE;}
      (junction 55) -> (junction 56) [order 1] : [VSCP_TimeTPdelay_s >= KSCP_DelayECDTandECDT_s]
      (junction 55) -> (junction 57) [order 2] : {VSCP_TimeTPdelay_s += task_time;}
      (junction 56) -> (junction 58) : {VSCP_TpDelayDone_flg = TRUE;}
      (junction 58) -> (junction 57)
    state Tirgger_ECDT3_and_Delay
      en: trigger_DT = TRUE;
      (default) -> (junction 123) : {
          |  VSCP_TpDelayDone_flg = FALSE;
          |  VSCP_TimeTPdelay_s = 0;}
      Tirgger_ECDT3_and_Delay -> (junction 123) [order 1] : {trigger_DT = FALSE;}
      (junction 123) -> (junction 124) [order 1] : [VSCP_TimeTPdelay_s >= KSCP_DelayECDTandECDT_s]
      (junction 123) -> (junction 125) [order 2] : {VSCP_TimeTPdelay_s += task_time;}
      (junction 124) -> (junction 126) : {VSCP_TpDelayDone_flg = TRUE;}
      (junction 126) -> (junction 125)
    state Tirgger_ECDT4_and_Delay
      en: trigger_DT = TRUE;
      (default) -> (junction 134) : {
          |  VSCP_TpDelayDone_flg = FALSE;
          |  VSCP_TimeTPdelay_s = 0;}
      Tirgger_ECDT4_and_Delay -> (junction 134) [order 1] : {trigger_DT = FALSE;}
      (junction 134) -> (junction 135) [order 1] : [VSCP_TimeTPdelay_s >= KSCP_DelayECDTandECDT_s]
      (junction 134) -> (junction 136) [order 2] : {VSCP_TimeTPdelay_s += task_time;}
      (junction 135) -> (junction 137) : {VSCP_TpDelayDone_flg = TRUE;}
      (junction 137) -> (junction 136)
    state Tirgger_ECDT5_and_Delay
      en: trigger_DT = TRUE;
      (default) -> (junction 145) : {
          |  VSCP_TpDelayDone_flg = FALSE;
          |  VSCP_TimeTPdelay_s = 0;}
      Tirgger_ECDT5_and_Delay -> (junction 145) [order 1] : {trigger_DT = FALSE;}
      (junction 145) -> (junction 146) [order 1] : [VSCP_TimeTPdelay_s >= KSCP_DelayECDTandECDT_s]
      (junction 145) -> (junction 147) [order 2] : {VSCP_TimeTPdelay_s += task_time;}
      (junction 146) -> (junction 148) : {VSCP_TpDelayDone_flg = TRUE;}
      (junction 148) -> (junction 147)
    state Tirgger_ECDT6_and_Delay
      en: trigger_DT = TRUE;
      (default) -> (junction 156) : {
          |  VSCP_TpDelayDone_flg = FALSE;
          |  VSCP_TimeTPdelay_s = 0;}
      Tirgger_ECDT6_and_Delay -> (junction 156) [order 1] : {trigger_DT = FALSE;}
      (junction 156) -> (junction 157) [order 1] : [VSCP_TimeTPdelay_s >= KSCP_DelayECDTandRCBAM_s]
      (junction 156) -> (junction 158) [order 2] : {VSCP_TimeTPdelay_s += task_time;}
      (junction 157) -> (junction 159) : {VSCP_TpDelayDone_flg = TRUE;}
      (junction 159) -> (junction 158)
    state Trigger_RCBAM_and_Delay
      en: trigger_BAM = TRUE;
      (default) -> (junction 67) : {
          |  VSCP_TpDelayDone_flg = FALSE;
          |  VSCP_TimeTPdelay_s = 0;}
      Trigger_RCBAM_and_Delay -> (junction 67) [order 1] : {trigger_BAM = FALSE;}
      (junction 67) -> (junction 68) [order 1] : [VSCP_TimeTPdelay_s >= KSCP_DelayRCBAMandRCDT_s]
      (junction 67) -> (junction 69) [order 2] : {VSCP_TimeTPdelay_s += task_time;}
      (junction 68) -> (junction 70) : {VSCP_TpDelayDone_flg = TRUE;}
      (junction 70) -> (junction 69)
    state Tirgger_RCDT1_and_Delay
      en: trigger_DT = TRUE;
      (default) -> (junction 79) : {
          |  VSCP_TpDelayDone_flg = FALSE;
          |  VSCP_TimeTPdelay_s = 0;}
      Tirgger_RCDT1_and_Delay -> (junction 79) [order 1] : {trigger_DT = FALSE;}
      (junction 79) -> (junction 80) [order 1] : [VSCP_TimeTPdelay_s >= KSCP_DelayRCDTandRCDT_s]
      (junction 79) -> (junction 81) [order 2] : {VSCP_TimeTPdelay_s += task_time;}
      (junction 80) -> (junction 82) : {VSCP_TpDelayDone_flg = TRUE;}
      (junction 82) -> (junction 81)
    state Tirgger_RCDT2_and_Delay
      en: trigger_DT = TRUE;
      (default) -> (junction 300) : {
          |  VSCP_TpDelayDone_flg = FALSE;
          |  VSCP_TimeTPdelay_s = 0;}
      Tirgger_RCDT2_and_Delay -> (junction 300) [order 1] : {trigger_DT = FALSE;}
      (junction 300) -> (junction 301) [order 1] : [VSCP_TimeTPdelay_s >= KSCP_DelayRCDTandRCDT_s]
      (junction 300) -> (junction 302) [order 2] : {VSCP_TimeTPdelay_s += task_time;}
      (junction 301) -> (junction 303) : {VSCP_TpDelayDone_flg = TRUE;}
      (junction 303) -> (junction 302)
    state Tirgger_RCDT3_and_Delay
      en: trigger_DT = TRUE;
      (default) -> (junction 311) : {
          |  VSCP_TpDelayDone_flg = FALSE;
          |  VSCP_TimeTPdelay_s = 0;}
      Tirgger_RCDT3_and_Delay -> (junction 311) [order 1] : {trigger_DT = FALSE;}
      (junction 311) -> (junction 312) [order 1] : [VSCP_TimeTPdelay_s >= KSCP_DelayRCDTandECBAM_s]
      (junction 311) -> (junction 313) [order 2] : {VSCP_TimeTPdelay_s += task_time;}
      (junction 312) -> (junction 314) : {VSCP_TpDelayDone_flg = TRUE;}
      (junction 314) -> (junction 313)
    (default) -> (junction 3)
    (junction 119) -> (junction 3)
    (junction 117) -> (junction 119)
    (junction 3) -> Trigger_ECBAM_and_Delay : { VSCP_CFGEM1Ctrl_raw = 0x20;
        |   VSCP_CFGEM1BAMTSize_raw = 0x27;
        |   VSCP_CFGEM1BAMTNum_raw = 0x06;
        |   VSCP_CFGEM1BAMRsv_raw = 0xFF;
        |   VSCP_CFGEM1BAMPGN_raw = 0xFEE3;}
    Trigger_ECBAM_and_Delay -> Tirgger_ECDT1_and_Delay [order 1] : [VSCP_TpDelayDone_flg]
        | {VSCP_DTbyte0_raw = 0x01; VSCP_DTbyte1_raw = 0xFF; VSCP_DTbyte2_raw = 0xFF; VSCP_DTbyte3_raw = 0xFF;
        |  VSCP_DTbyte4_raw = 0xFF; VSCP_DTbyte5_raw = 0xFF; VSCP_DTbyte6_raw = 0xFF; VSCP_DTbyte7_raw = 0xFF;}
    Tirgger_ECDT1_and_Delay -> Tirgger_ECDT2_and_Delay [order 1] : [VSCP_TpDelayDone_flg]
        | {VSCP_DTbyte0_raw = 0x02; VSCP_DTbyte1_raw = 0xFF; VSCP_DTbyte2_raw = 0xFF; VSCP_DTbyte3_raw = 0xFF;
        |  VSCP_DTbyte4_raw = 0xFF; VSCP_DTbyte5_raw = 0xFF; VSCP_DTbyte6_raw = 0xFF; VSCP_DTbyte7_raw = 0xFF;}
    Tirgger_ECDT2_and_Delay -> Tirgger_ECDT3_and_Delay [order 1] : [VSCP_TpDelayDone_flg]
        | {VSCP_DTbyte0_raw = 0x03; VSCP_DTbyte1_raw = 0xFF; VSCP_DTbyte2_raw = 0xFF; VSCP_DTbyte3_raw = 0xFF;
        |  VSCP_DTbyte4_raw = 0xFF; VSCP_DTbyte5_raw = 0xFF; VSCP_DTbyte6_raw = VSCP_ECDTbyte6_raw; VSCP_DTbyte7_raw = VSCP_ECDTbyte7_raw;}
    Tirgger_ECDT3_and_Delay -> Tirgger_ECDT4_and_Delay [order 1] : [VSCP_TpDelayDone_flg]
        | {VSCP_DTbyte0_raw = 0x04; VSCP_DTbyte1_raw = 0xFF; VSCP_DTbyte2_raw = 0xFF; VSCP_DTbyte3_raw = 0xFF;
        |  VSCP_DTbyte4_raw = 0xFF; VSCP_DTbyte5_raw = 0xFF; VSCP_DTbyte6_raw = 0xFF; VSCP_DTbyte7_raw = 0xFF;}
    Tirgger_ECDT4_and_Delay -> Tirgger_ECDT5_and_Delay [order 1] : [VSCP_TpDelayDone_flg]
        | {VSCP_DTbyte0_raw = 0x05; VSCP_DTbyte1_raw = 0xFF; VSCP_DTbyte2_raw = 0xFF; VSCP_DTbyte3_raw = 0xFF;
        |  VSCP_DTbyte4_raw = 0xFF; VSCP_DTbyte5_raw = 0xFF; VSCP_DTbyte6_raw = 0xFF; VSCP_DTbyte7_raw = 0xFF;}
    Tirgger_ECDT5_and_Delay -> Tirgger_ECDT6_and_Delay [order 1] : [VSCP_TpDelayDone_flg]
        | {VSCP_DTbyte0_raw = 0x06; VSCP_DTbyte1_raw = 0xFF; VSCP_DTbyte2_raw = 0xFF; VSCP_DTbyte3_raw = 0xFF;
        |  VSCP_DTbyte4_raw = 0xFF; VSCP_DTbyte5_raw = 0xFF; VSCP_DTbyte6_raw = 0xFF; VSCP_DTbyte7_raw = 0xFF;}
    Tirgger_ECDT6_and_Delay -> Trigger_RCBAM_and_Delay [order 1] : [VSCP_TpDelayDone_flg]
        | { VSCP_CFGEM1Ctrl_raw = 0x20;
        |   VSCP_CFGEM1BAMTSize_raw = 0x13;
        |   VSCP_CFGEM1BAMTNum_raw = 0x03;
        |   VSCP_CFGEM1BAMRsv_raw = 0xFF;
        |   VSCP_CFGEM1BAMPGN_raw = 0xFEE1;}
    Trigger_RCBAM_and_Delay -> Tirgger_RCDT1_and_Delay [order 1] : [VSCP_TpDelayDone_flg]
        | {VSCP_DTbyte0_raw = 0x01; VSCP_DTbyte1_raw = 0x40; VSCP_DTbyte2_raw = 0xFF; VSCP_DTbyte3_raw = 0xFF;
        |  VSCP_DTbyte4_raw = 0xFF; VSCP_DTbyte5_raw = 0xFF; VSCP_DTbyte6_raw = 0xFF; VSCP_DTbyte7_raw = 0xFF;}
    Tirgger_RCDT1_and_Delay -> Tirgger_RCDT2_and_Delay [order 1] : [VSCP_TpDelayDone_flg]
        | {VSCP_DTbyte0_raw = 0x02; VSCP_DTbyte1_raw = 0xFF; VSCP_DTbyte2_raw = 0xFF; VSCP_DTbyte3_raw = 0xFF;
        |  VSCP_DTbyte4_raw = 0xFF; VSCP_DTbyte5_raw = 0xFF; VSCP_DTbyte6_raw = 0xFF; VSCP_DTbyte7_raw = 0xFF;}
    Tirgger_RCDT2_and_Delay -> Tirgger_RCDT3_and_Delay [order 1] : [VSCP_TpDelayDone_flg]
        | {VSCP_DTbyte0_raw = 0x03; VSCP_DTbyte1_raw = 0xFF; VSCP_DTbyte2_raw = 0xFF; VSCP_DTbyte3_raw = VSCP_RCDTbyte3_raw;
        |  VSCP_DTbyte4_raw = VSCP_RCDTbyte4_raw; VSCP_DTbyte5_raw = 0xFF; VSCP_DTbyte6_raw = 0xFF; VSCP_DTbyte7_raw = 0xFF;}
    Tirgger_RCDT3_and_Delay -> (junction 115) [order 1] : [VSCP_TpDelayDone_flg]
    (junction 115) -> (junction 117)
  (default) -> TP
  data: task_time input; KSCP_DelayECBAMandECDT_s input; KSCP_DelayECDTandECDT_s input; KSCP_DelayECDTandRCBAM_s input; trigger_BAM output boolean; VSCP_CFGEM1Ctrl_raw output uint8; VSCP_CFGEM1BAMTSize_raw output uint16; VSCP_CFGEM1BAMTNum_raw output uint8; VSCP_CFGEM1BAMRsv_raw output uint8; VSCP_CFGEM1BAMPGN_raw output uint32; trigger_DT output boolean; VSCP_TimeTPdelay_s local single; TRUE parameter; FALSE parameter; VSCP_TpDelayDone_flg local boolean; KSCP_DelayRCBAMandRCDT_s input; KSCP_DelayRCDTandRCDT_s input; KSCP_DelayRCDTandECBAM_s input; VSCP_DTbyte0_raw output uint8; VSCP_DTbyte1_raw output uint8; VSCP_DTbyte2_raw output uint8; VSCP_DTbyte3_raw output uint8; VSCP_DTbyte4_raw output uint8; VSCP_DTbyte5_raw output uint8; VSCP_DTbyte6_raw output uint8; VSCP_DTbyte7_raw output uint8; VSCP_ECDTbyte6_raw input; VSCP_ECDTbyte7_raw input; VSCP_RCDTbyte3_raw input; VSCP_RCDTbyte4_raw input
